simulink model "Final_kalman_filter_observer_LQG"  (R2024a)
settings: Solver=VariableStepAuto  StartTime=0.0  StopTime=10.0  RelTol=1e-3
undefined symbols (not defined in the file): A_aug, A_obs, B_aug, B_obs, C_aug, C_obs, D_aug, D_obs, disturbance, g_val, Ki, Kx, m_val, Noise_vector, r_pos, x0
libraries: simulink x1
settings Model: Creator=yufon  LastModifiedBy=yufon

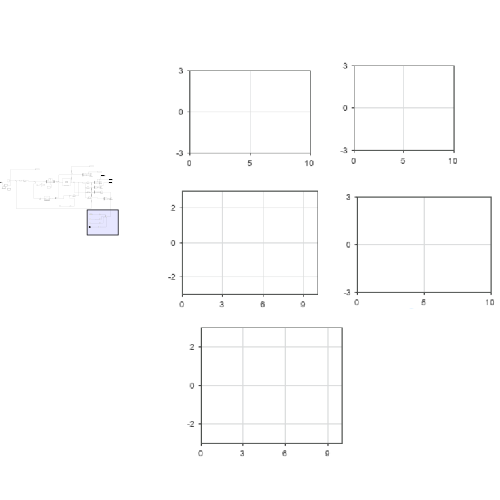
[thumbnail: Simulink's stored preview of the top-level diagram]
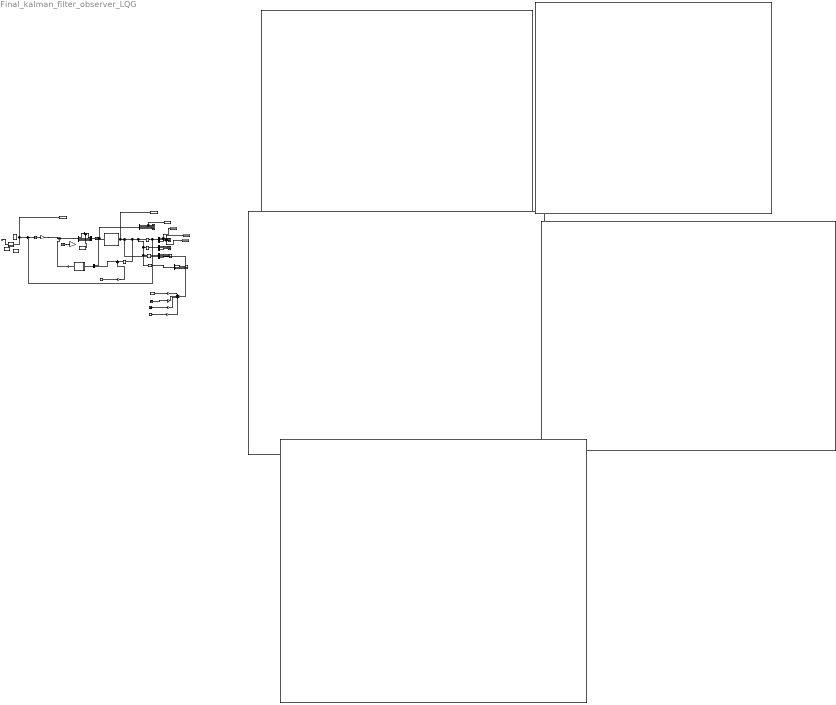
== system Final_kalman_filter_observer_LQG ==
  note: Wind and Other Pertubations
  Band-Limited White Noise : simulink/Sources/Band-Limited White Noise  Cov=[0.001]  Ts=0.1  seed=[23341]
  Body Abgular Selector : Selector  InputPortWidth=12  IndexOptions=Index vector (dialog)  Indices=[10 11 12]  OutputSizes=1
  Body Abgular Selector1 : Selector  InputPortWidth=12  IndexOptions=Index vector (dialog)  Indices=[7 8 9]  OutputSizes=1
  Body Linear Velocities : Scope  NumInputPorts=3
  Circular Trajectory1 : MATLAB Function  TreatAsAtomicUnit=on
  Clock : Clock
  Constant1 : Constant  Value=r_pos  VectorParams1D=off
  Constant3 : Constant  Value=m_val*g_val
  Control Input Scope : Scope  NumInputPorts=4
  Dashboard Scope{,1..4} (5 alike) : DashboardScope
  Demux{,1,3,5} (4 alike) : Demux  Outputs=3
  Demux2 : Demux
  Demux6 : Demux
  Display : Display
  Display1 : Display
  Display2 : Display
  Gain{,1..2,4} (4 alike) : Gain  Gain=0
  Gain3 : Gain  Gain=m_val*g_val
  Gain5 : Gain  Gain=Noise_vector
  Integrator Gain : Gain  Gain=Ki  Multiplication=Matrix(K*u)
  Integrator3 : Integrator
  KALMAN FILTER : Subsystem
  LQR Gain : Gain  Gain=Kx  Multiplication=Matrix(K*u)
  Linearised Qaudrotor Model : StateSpace  A=A_aug  B=B_aug  C=C_aug  D=D_aug  InitialCondition=0
  MATLAB Function1 : MATLAB Function  TreatAsAtomicUnit=on
  MATLAB Function2 : MATLAB Function  TreatAsAtomicUnit=on
  Mux1 : Mux  Inputs=2
  Mux2 : Mux
  Orientation Scope : Scope  NumInputPorts=3
  Orientation Selector1 : Selector  InputPortWidth=12  IndexOptions=Index vector (dialog)  Indices=[4 5 6]  OutputSizes=1
  Position Scope : Scope  NumInputPorts=3
  Position Scope1 : Scope  NumInputPorts=3
  Position Selector : Selector  InputPortWidth=12  IndexOptions=Index vector (dialog)  Indices=[1 2 3]  OutputSizes=1
  Position Selector1 : Selector  InputPortWidth=12  IndexOptions=Index vector (dialog)  Indices=[1 2 3 4 5 6]  OutputSizes=1
  Pulse Generator1 : DiscretePulseGenerator  PulseType=Time based  Period=10  PulseWidth=20  PhaseDelay=5
  Random Number : RandomNumber  Variance=0.5  SampleTime=0.1
  Saturation1 : Saturate  UpperLimit=[30; 0.15; 0.1; 0.5]  LowerLimit=[-3; -0.15; -0.1; -0.5]
  Sine Wave : Sin  Frequency=0.5  SampleTime=0
  Step : Step  Before=zeros(12,1)  After=disturbance  SampleTime=0
  Step1 : Step  Time=10  Before=1  After=1.25  SampleTime=0
  Sum : Sum  Inputs=|--
  Sum1 : Sum  Inputs=|+-
  Sum2 : Sum  Inputs=|++++
  Sum3 : Sum  Inputs=|++
  Sum4 : Sum  Inputs=|++
  Sum5 : Sum  Inputs=|++
  To Workspace : ToWorkspace  VariableName=X_states  SampleTime=-1
  To Workspace1 : ToWorkspace  VariableName=U1  SaveFormat=Timeseries  SampleTime=-1
  To Workspace2 : ToWorkspace  VariableName=r_traj  SaveFormat=Timeseries  SampleTime=-1
  wires:
  Gain5/1 -> Sum5/2
  Band-Limited White Noise/1 -> Gain5/1
  Saturation1/1 -> Mux1/1, Demux2/1, Linearised Qaudrotor Model/1
  Demux/3 -> Display1/1, Position Scope/3  "Z"
  Position Selector1/1 -> Sum5/1
  Demux3/2 -> Position Scope1/2  "q"
  Demux6/3 -> Mux2/3  "U3"
  Demux/2 -> Display/1, Position Scope/2  "Y"
  Body Abgular Selector/1 -> Demux3/1
  Demux2/1 -> To Workspace1/1, Control Input Scope/1  "U1"
  LQR Gain/1 -> Sum/2
  Sum4/1 -> Position Selector1/1, Body Abgular Selector1/1, Body Abgular Selector/1, Orientation Selector1/1, Position Selector/1
  Clock/1 -> MATLAB Function1/1(t)
  Position Selector/1 -> Demux/1, Sum1/2
  Sum1/1 -> Integrator3/1
  Demux3/1 -> Position Scope1/1  "p"
  Demux2/2 -> Control Input Scope/2  "U2"
  Demux3/3 -> Position Scope1/3  "r"
  Demux6/2 -> Mux2/2  "U2"
  Demux6/1 -> Sum3/1  "U1"
  Demux5/1 -> Body Linear Velocities/1  "u"
  Sum5/1 -> Mux1/2
  Demux6/4 -> Mux2/4  "U4"
  Orientation Selector1/1 -> Demux1/1
  Demux2/3 -> Control Input Scope/3  "U3"
  Demux/1 -> Display2/1, Position Scope/1  "X"
  Demux5/3 -> Body Linear Velocities/3  "w"
  Demux5/2 -> Body Linear Velocities/2  "u"
  Gain2/1 -> Sum2/1
  Demux2/4 -> Control Input Scope/4  "U4"
  Sum2/1 -> Sum4/2
  Sum/1 -> Demux6/1
  Demux1/3 -> Orientation Scope/3  "Psi"
  Mux2/1 -> Saturation1/1
  Pulse Generator1/1 -> Gain4/1
  Body Abgular Selector1/1 -> Demux5/1
  MATLAB Function1/1(r) -> To Workspace2/1, Sum1/1
  Random Number/1 -> Gain2/1
  Integrator3/1 -> Integrator Gain/1
  KALMAN FILTER/1(X_state) -> LQR Gain/1
  Gain4/1 -> Sum2/4
  Sine Wave/1 -> Gain/1
  Constant3/1 -> Sum3/2
  Mux1/1 -> KALMAN FILTER/1(In1)
  Integrator Gain/1 -> Sum/1
  Gain/1 -> Sum2/3
  Sum3/1 -> Mux2/1
  Gain1/1 -> Sum2/2
  Demux1/2 -> Orientation Scope/2  "Thata"
  Linearised Qaudrotor Model/1 -> Sum4/1, To Workspace/1  "X_state"
  Step/1 -> Gain1/1
  Step1/1 -> Gain3/1
  Demux1/1 -> Orientation Scope/1  "Phi"

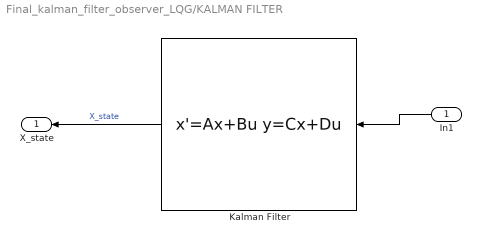
== system Final_kalman_filter_observer_LQG/KALMAN FILTER ==
  In1 : Inport
  Kalman Filter : StateSpace  A=A_obs  B=B_obs  C=C_obs  D=D_obs  InitialCondition=x0
  X_state : Outport
  wires:
  Kalman Filter/1 -> X_state/1  "X_state"
  In1/1 -> Kalman Filter/1

== matlab function Final_kalman_filter_observer_LQG/Circular Trajectory1 ==
  data: t input; r output


function r = trajectory(t)

% Parameters (you can also pass these in or make them tunable)
R = 5;           % Radius of circle (meters)
omega = 0.1;     % Angular frequency (rad/s)
z0 = 10;         % Base altitude (meters)
A = 2;           % Amplitude of vertical oscillation (meters)
omega_z = 0.05;  % Vertical oscillation frequency (rad/s)

% Reference trajectory components
r_x = R * cos(omega * t);
r_y = R * sin(omega * t);
r_z = z0 + A * sin(omega_z * t);  % Set A = 0 for pure circle

% Output as a 3x1 vector
r = [r_x; r_y; r_z];

== matlab function Final_kalman_filter_observer_LQG/MATLAB Function1 ==
  data: t input; r output
function r = rect_trajectory(t)

% Parameters
L = 10;        % Length of rectangle (x-direction)
W = 5;         % Width of rectangle (y-direction)
z0 = 10;       % Fixed height
T_side = 5;    % Time to complete one side
T_cycle = 4 * T_side;

% Normalize time to current phase
t_mod = mod(t, T_cycle);

% Initialize reference
x = 0;
y = 0;

if t_mod < T_side
    % Move right (+x)
    x = L * (t_mod / T_side);
    y = 0;

elseif t_mod < 2*T_side
    % Move forward (+y)
    x = L;
    y = W * ((t_mod - T_side) / T_side);

elseif t_mod < 3*T_side
    % Move left (−x)
    x = L - L * ((t_mod - 2*T_side) / T_side);
    y = W;

else
    % Move backward (−y)
    x = 0;
    y = W - W * ((t_mod - 3*T_side) / T_side);
end

% Fixed height
z = z0;

% Output as column vector
r = [x; y; z];

== matlab function Final_kalman_filter_observer_LQG/MATLAB Function2 ==
  data: t input; r output
function r = rect_trajectory(t)

% Parameters
L = 10;        % Length of rectangle (x-direction)
W = 5;         % Width of rectangle (y-direction)
z0 = 10;       % Fixed height
T_side = 5;    % Time to complete one side
T_cycle = 4 * T_side;

% Normalize time to current phase
t_mod = mod(t, T_cycle);

% Initialize reference
x = 0;
y = 0;

if t_mod < T_side
    % Move right (+x)
    x = L * (t_mod / T_side);
    y = 0;

elseif t_mod < 2*T_side
    % Move forward (+y)
    x = L;
    y = W * ((t_mod - T_side) / T_side);

elseif t_mod < 3*T_side
    % Move left (−x)
    x = L - L * ((t_mod - 2*T_side) / T_side);
    y = W;

else
    % Move backward (−y)
    x = 0;
    y = W - W * ((t_mod - 3*T_side) / T_side);
end

% Fixed height
z = z0;

% Output as column vector
r = [x; y; z];
